simulink model "mdaqdemo_uart"  (R2013a)
settings: Solver=FixedStepDiscrete  SolverMode=SingleTasking  StartTime=0.0  StopTime=10.0  RelTol=1e-3
libraries: microdaq_lib x5, etargetslib x2, simulink x1
settings Model: Creator=skibool  LastModifiedBy=skibool
settings OptimizationCC: OptimizeModelRefInitCode=on  LifeSpan=1
settings DebuggingCC: UnderspecifiedInitializationDetection=Simplified  StateNameClashWarn=none
settings HardwareCC: ProdBitPerLong=40  ProdLargestAtomicInteger=Integer  ProdIntDivRoundTo=Zero  ProdEndianess=LittleEndian  ProdHWDeviceType=Texas Instruments->C6000
settings RTWCC: SystemTargetFile=microdaq.tlc  TemplateMakefile=microdaq.tmf  PostCodeGenCommand=microdaq_postcodegen(buildInfo)  Description=MicroDAQ Real-Time Measurement System  ProcessScript=microdaq_make_rtw_hook
settings CodeAppCC: IgnoreCustomStorageClasses=off
settings STFCustomTargetCC: CodeReplacementLibrary=TI C674x  CombineOutputUpdateFcns=on  ERTCustomFileBanners=on  SupportContinuousTime=off  SupportNonInlinedSFcns=off  MATLABClassNameForMDSCustomization=Simulink.SoftwareTarget.ERTCustomization  SystemTargetFile=microdaq.tlc
settings ERTTargetCC: CodeReplacementLibrary=TI C674x  GenerateSampleERTMain=off  ParMdlRefBuildCompliant=off  CompOptLevelCompliant=off  ConcurrentExecutionCompliant=off  ERTFirstTimeCompliant=off  ModelStepFunctionPrototypeControlCompliant=off  CPPClassGenCompliant=off  ExtModeStaticAlloc=on  ExtModeStaticAllocSize=10485760  ExtModeMexArgs=getpref('microdaq','TargetIP') 1 4344  ERTCustomFileTemplate=microdaq_main.tlc

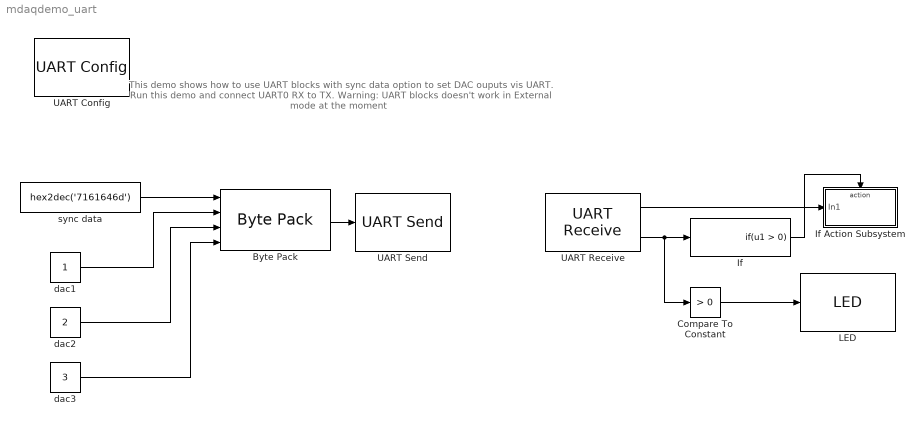
== system mdaqdemo_uart ==
  note: This demo shows how to use UART blocks with sync
      | data option to set DAC ouputs vis UART.
      |
      | Run this demo and connect UART0 RX to TX.
      |
      | Warning: UART blocks doesn't work in External mode at the moment
  Byte Pack : etargetslib/Byte Pack  datatypes={'uint32','single','single','single'}  byteAlign=1
  Compare To Constant : simulink/Logic and Bit Operations/Compare To Constant  relop=>  const=0  OutDataTypeStr=uint8
  If : If  ShowElse=off
  If Action Subsystem : Subsystem  TreatAsAtomicUnit=on
  LED : microdaq_lib/LED  SParameter1=D1
  UART Config : microdaq_lib/UART Config  pModule=UART0  pBaudRate=115200  pDataBits=8  pParity=None  pStopBits=1  pFlowControl=None
  UART Receive : microdaq_lib/UART Receive  pModule=UART0  pDataSize=12  pUseHeader=on  pHeaderStr=7161646d  pHeader=0  pBlocking=off  pTimeout=100  SampleTime=0.1
  UART Send : microdaq_lib/UART Send  pModule=UART0  pDataSize=16  SampleTime=1
  dac1 : Constant  OutDataTypeStr=single
  dac2 : Constant  Value=2  OutDataTypeStr=single
  dac3 : Constant  Value=3  OutDataTypeStr=single
  sync data : Constant  Value=hex2dec('7161646d')  OutDataTypeStr=uint32
  wires:
  If/1 -> If Action Subsystem/Action
  UART Receive/2 -> Compare To Constant/1, If/1
  UART Receive/1 -> If Action Subsystem/1(In1)
  sync data/1 -> Byte Pack/1
  dac1/1 -> Byte Pack/2
  dac2/1 -> Byte Pack/3
  dac3/1 -> Byte Pack/4
  Byte Pack/1 -> UART Send/1
  Compare To Constant/1 -> LED/1

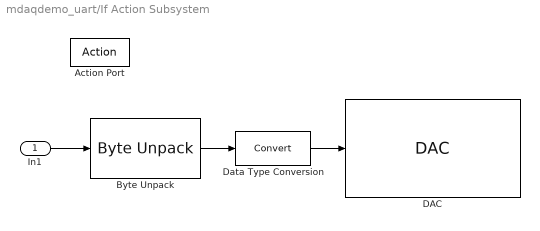
== system mdaqdemo_uart/If Action Subsystem ==
  In1 : Inport
  Action Port : ActionPort  ActionType=then
  Byte Unpack : etargetslib/Byte Unpack  dimensions={[3]}  datatypes={'single'}  byteAlign=1
  DAC : microdaq_lib/DAC  pConverter=DAC01 - 8 channel, 12-bit, 0-5V range  pChannel=[ 1 2 3]  pChannelCount=ones([1 1 ])  pMode=Sequential  pModeTrig=Software  pTermAll=on  pTerm=0.0  SampleTime=-1
  Data Type Conversion : DataTypeConversion
  wires:
  In1/1 -> Byte Unpack/1
  Byte Unpack/1 -> Data Type Conversion/1
  Data Type Conversion/1 -> DAC/1
